simulink model "Q1_M3"  (R2024b)
settings: Solver=VariableStepAuto  StartTime=0.0  StopTime=10.0  RelTol=1e-3
model workspace (MAT data in the model file):
  b1 = 50
  b2 = 70
  k1 = 400
  k2 = 600
  m = 10
settings Model: Creator=chall  LastModifiedBy=chall

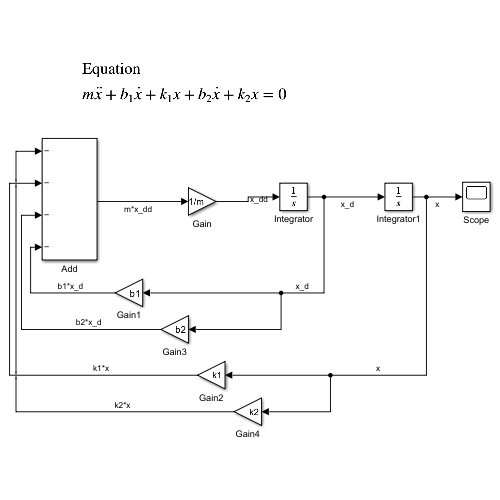
[thumbnail: Simulink's stored preview of the top-level diagram]
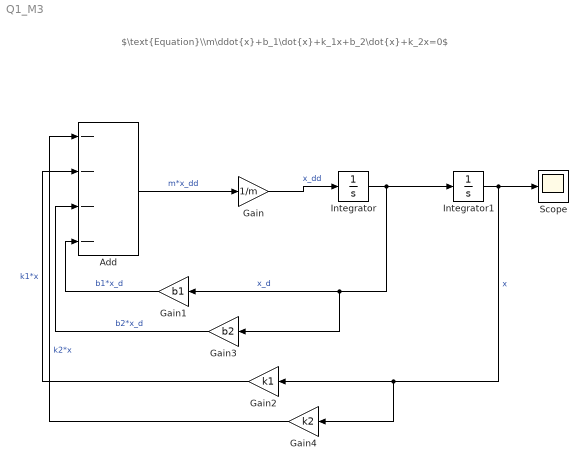
== system Q1_M3 ==
  note: $\text{Equation}\\m\ddot{x}+b_1\dot{x}+k_1x+b_2\dot{x}+k_2x=0$
  Add : Sum  Inputs=----
  Gain : Gain  Gain=1/m
  Gain1 : Gain  Gain=b1
  Gain2 : Gain  Gain=k1
  Gain3 : Gain  Gain=b2
  Gain4 : Gain  Gain=k2
  Integrator : Integrator
  Integrator1 : Integrator  InitialCondition=0.8
  Scope : Scope
  wires:
  Add/1 -> Gain/1  "m*x_dd"
  Gain/1 -> Integrator/1  "x_dd"
  Integrator/1 -> Gain3/1, Gain1/1, Integrator1/1  "x_d"
  Integrator1/1 -> Gain4/1, Gain2/1, Scope/1  "x"
  Gain1/1 -> Add/4  "b1*x_d"
  Gain3/1 -> Add/3  "b2*x_d"
  Gain2/1 -> Add/2  "k1*x"
  Gain4/1 -> Add/1  "k2*x"
